simulink model "pmsm_quad_pcie"  (R2020b)
settings: Solver=FixedStepDiscrete  StartTime=0.0  StopTime=5  FixedStep=1e-3  RelTol=1e-3
PostLoadFcn:
  | try
  | cell = struct2cell(dir(fullfile(speedgoatroot_hdlb, 'hdlsrc', 'quadrature', '*.vhd')));
  | addSourceFiles = strjoin(fullfile(cell(2,:),cell(1,:)), ';');
  | hdlset_param('quadrature_example_hdlc/DUT Quadrature', 'IPCoreAdditionalFiles', addSourceFiles);
  | end
libraries: simulink x2, quadrature_fpgalib x1, quadrature_cpulib x1
settings Model: ModifiedByFormat=Speedgoat GmbH  Creator=Speedgoat GmbH  LastModifiedBy=Speedgoat GmbH
settings DataIOCC: ReturnWorkspaceOutputs=off
settings OptimizationCC: BlockReduction=off  ConditionallyExecuteInputs=off  DefaultParameterBehavior=Inlined
settings DebuggingCC: AlgebraicLoopMsg=error  ParameterOverflowMsg=warning  PregeneratedLibrarySubsystemCodeDiagnostic=none  ArithmeticOperatorsInVariantConditions=warning
settings HardwareCC: ProdBitPerPointer=32  ProdBitPerSizeT=32  ProdBitPerPtrDiffT=32  ProdLargestAtomicFloat=None  ProdIntDivRoundTo=Undefined  ProdEndianess=Unspecified  ProdWordSize=32  ProdHWDeviceType=ASIC/FPGA->ASIC/FPGA  TargetBitPerPointer=64  TargetBitPerSizeT=64  TargetBitPerPtrDiffT=64  TargetLongLongMode=on  TargetIntDivRoundTo=Zero  TargetEndianess=LittleEndian  TargetWordSize=64  TargetHWDeviceType=Custom Processor->MATLAB Host Computer  ProdEqTarget=off
settings SFSimCC: SimUseLocalCustomCode=off  CustomCodeUndefinedFunction=UseInterfaceOnly
settings RTWCC: RTWUseLocalCustomCode=off

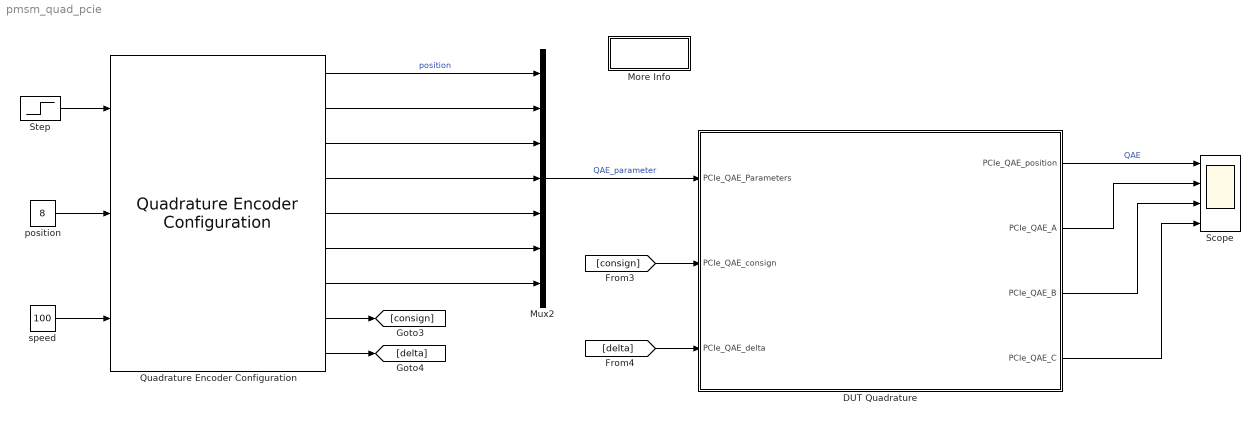
== system pmsm_quad_pcie ==
  DUT Quadrature : Subsystem
  More Info : Subsystem
      settings: OpenFcn=|
      | try
      | speedgoat.hdlioblockset.doc('page', 'quadrature');
      | catch
      | web('https://www.speedgoat.com/help/hdlcoder/page/hdlb/refentry_hdl_blockset_quadrature');
      | end
      mask Display: disp('Documentation')
  Mux2 : Mux  Inputs=7
  Quadrature Encoder Configuration : quadrature_cpulib/Quadrature Encoder Configuration  fpgaFreq=100e6  n_channels=1  numSeg=[16]  phaseAngle=90  initPos=[0]  freeWheel=on
      settings: SourceProductName=Simulink Real-Time: Speedgoat HDL Blockset
  Scope : Scope  NumInputPorts=4
  Step : Step  Time=0.002
  position : Constant  Value=8  SampleTime=-1
  speed : Constant  Value=100  SampleTime=-1
  wires:
  position/1 -> Quadrature Encoder Configuration/2
  speed/1 -> Quadrature Encoder Configuration/3
  Quadrature Encoder Configuration/2 -> Mux2/2
  Quadrature Encoder Configuration/3 -> Mux2/3
  Quadrature Encoder Configuration/6 -> Mux2/6
  Quadrature Encoder Configuration/7 -> Mux2/7
  Quadrature Encoder Configuration/8 -> [consign]
  Quadrature Encoder Configuration/9 -> [delta]
  Mux2/1 -> DUT Quadrature/1(PCIe_QAE_Parameters)  "QAE_parameter"
  Quadrature Encoder Configuration/1 -> Mux2/1  "position"
  Quadrature Encoder Configuration/4 -> Mux2/4
  [consign] -> DUT Quadrature/2(PCIe_QAE_consign)
  [delta] -> DUT Quadrature/3(PCIe_QAE_delta)
  Quadrature Encoder Configuration/5 -> Mux2/5
  DUT Quadrature/2(PCIe_QAE_A) -> Scope/2
  DUT Quadrature/3(PCIe_QAE_B) -> Scope/3
  DUT Quadrature/4(PCIe_QAE_C) -> Scope/4
  DUT Quadrature/1(PCIe_QAE_position) -> Scope/1  "QAE"
  Step/1 -> Quadrature Encoder Configuration/1

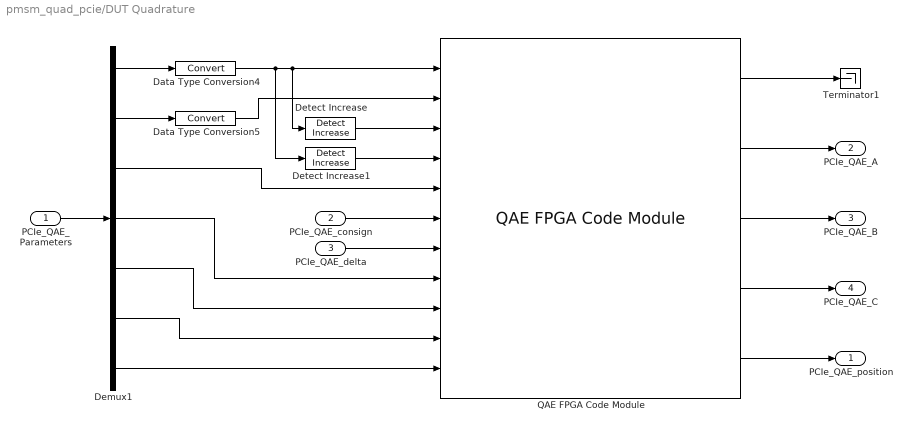
== system pmsm_quad_pcie/DUT Quadrature ==
  PCIe_QAE_Parameters : Inport
  PCIe_QAE_consign : Inport  Port=2  OutDataTypeStr=uint32  PortDimensions=1
  PCIe_QAE_delta : Inport  Port=3  PortDimensions=1
  Data Type Conversion4 : DataTypeConversion
  Data Type Conversion5 : DataTypeConversion
  Demux1 : Demux  Outputs=7
  Detect Increase : simulink/Logic and Bit Operations/Detect Increase  vinit=0.0  OutDataTypeStr=boolean
  Detect Increase1 : simulink/Logic and Bit Operations/Detect Increase  vinit=0.0  OutDataTypeStr=boolean
  QAE FPGA Code Module : quadrature_fpgalib/QAE FPGA Code Module  SystemSampleTime=-1  VariantActivationTime=update diagram  Latency=0  AutoFrameSizeCalculation=off
      settings: SourceProductName=Simulink Real-Time: Speedgoat Functionality Package
  Terminator1 : Terminator
  PCIe_QAE_position : Outport  VectorParamsAs1DForOutWhenUnconnected=off
  PCIe_QAE_A : Outport  Port=2  VectorParamsAs1DForOutWhenUnconnected=off
  PCIe_QAE_B : Outport  Port=3  VectorParamsAs1DForOutWhenUnconnected=off
  PCIe_QAE_C : Outport  Port=4  VectorParamsAs1DForOutWhenUnconnected=off
  wires:
  QAE FPGA Code Module/5 -> PCIe_QAE_position/1
  Detect Increase1/1 -> QAE FPGA Code Module/4
  Detect Increase/1 -> QAE FPGA Code Module/3
  QAE FPGA Code Module/4 -> PCIe_QAE_C/1
  QAE FPGA Code Module/2 -> PCIe_QAE_A/1
  QAE FPGA Code Module/3 -> PCIe_QAE_B/1
  PCIe_QAE_delta/1 -> QAE FPGA Code Module/7
  QAE FPGA Code Module/1 -> Terminator1/1
  PCIe_QAE_consign/1 -> QAE FPGA Code Module/6
  Demux1/1 -> Data Type Conversion4/1
  Demux1/2 -> Data Type Conversion5/1
  Demux1/3 -> QAE FPGA Code Module/5
  Demux1/4 -> QAE FPGA Code Module/8
  Demux1/5 -> QAE FPGA Code Module/9
  PCIe_QAE_Parameters/1 -> Demux1/1
  Data Type Conversion4/1 -> Detect Increase1/1, QAE FPGA Code Module/1, Detect Increase/1
  Data Type Conversion5/1 -> QAE FPGA Code Module/2
  Demux1/6 -> QAE FPGA Code Module/10
  Demux1/7 -> QAE FPGA Code Module/11

== system pmsm_quad_pcie/More Info ==
